simulink library "lithium_ion_battery"  (R2026a)
settings: Solver=VariableStepAuto
undefined symbols (not defined in the file): param, q1Kalman, q2Kalman, q3Kalman, rKalman, tc, ts_battery
libraries: nesl_utility x5, fl_lib x4, lithium_ion_cell_lib x1, simulink x1
settings Model: Creator=dbagn  LastModifiedBy=d.bagnara

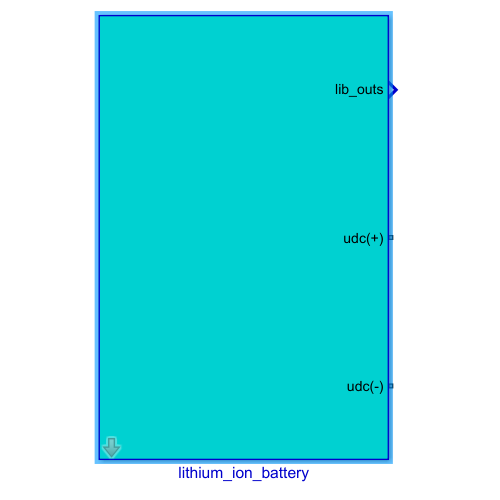
[thumbnail: Simulink's stored preview of the top-level diagram]
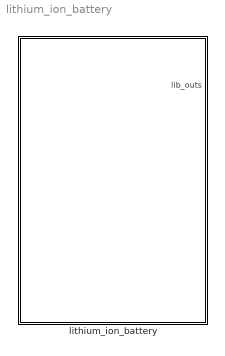
== system lithium_ion_battery ==
  lithium_ion_battery : Subsystem  mask{Q=50, number_of_cells=346, E_1=-1.031, E0=3.485, E1=0, E2=0, E3=0, Elog=-0.05, R0=0.0035, R1=0.0035, C1=0.5, M=125, alpha=35, soc_init=0.85, ts_battery=ts_battery, q1Kalman=q1Kalman, q2Kalman=q2Kalman, q3Kalman=q3Kalman, rKalman=rKalman, tc=tc, enable_white_noise_m=0, battery_voltage_init_m=param.battery.nominal_battery_voltage_1}
      mask prompts: Q "Nominal Charge Capacity (Ah)"; number_of_cells "Number of Cells"; E_1 "E_1 (V)"; E0 "E0 (V)"; E1 "E1 (V)"; E2 "E2 (V)"; E3 "E3 (V)"; Elog "Elog (V)"; R0 "R0 (Ohm)"; R1 "R1 (Ohm)"; C1 "C1 (F)"; M "Hysteresis coefficient (V)"; soc_init "State of Charge Init (pu)"; ts_battery "Sampling Time BESS"

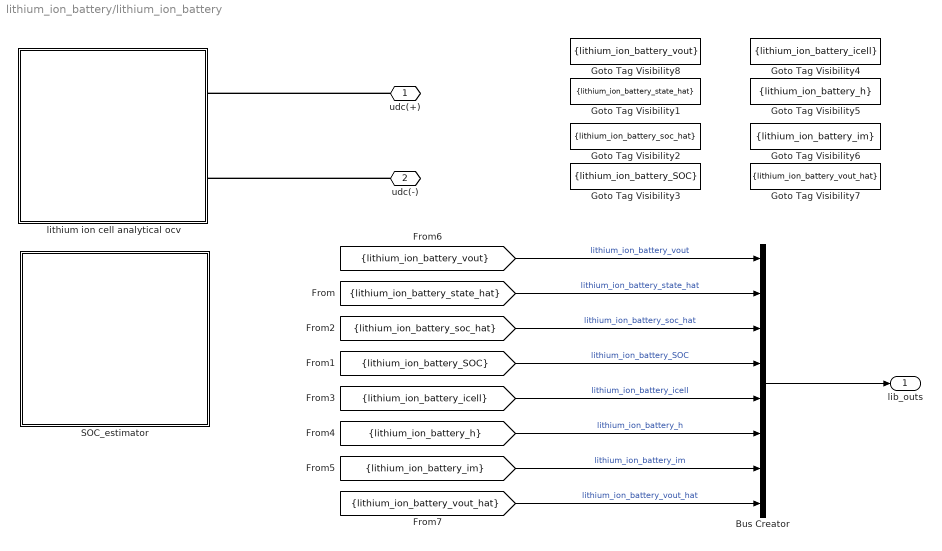
== system lithium_ion_battery/lithium_ion_battery ==
  Bus Creator : BusCreator  Inputs=8
  Goto Tag Visibility1 : GotoTagVisibility  GotoTag=lithium_ion_battery_state_hat
  Goto Tag Visibility2 : GotoTagVisibility  GotoTag=lithium_ion_battery_soc_hat
  Goto Tag Visibility3 : GotoTagVisibility  GotoTag=lithium_ion_battery_SOC
  Goto Tag Visibility4 : GotoTagVisibility  GotoTag=lithium_ion_battery_icell
  Goto Tag Visibility5 : GotoTagVisibility  GotoTag=lithium_ion_battery_h
  Goto Tag Visibility6 : GotoTagVisibility  GotoTag=lithium_ion_battery_im
  Goto Tag Visibility7 : GotoTagVisibility  GotoTag=lithium_ion_battery_vout_hat
  Goto Tag Visibility8 : GotoTagVisibility  GotoTag=lithium_ion_battery_vout
  SOC_estimator : Subsystem
  lithium ion cell analytical ocv : Subsystem
  udc(+) : PMIOPort  Side=Right
  udc(-) : PMIOPort  Port=2  Side=Right
  lib_outs : Outport
  wires:
  [lithium_ion_battery_im] -> Bus Creator/7  "lithium_ion_battery_im"
  [lithium_ion_battery_h] -> Bus Creator/6  "lithium_ion_battery_h"
  [lithium_ion_battery_icell] -> Bus Creator/5  "lithium_ion_battery_icell"
  [lithium_ion_battery_SOC] -> Bus Creator/4  "lithium_ion_battery_SOC"
  [lithium_ion_battery_soc_hat] -> Bus Creator/3  "lithium_ion_battery_soc_hat"
  [lithium_ion_battery_state_hat] -> Bus Creator/2  "lithium_ion_battery_state_hat"
  [lithium_ion_battery_vout] -> Bus Creator/1  "lithium_ion_battery_vout"
  Bus Creator/1 -> lib_outs/1
  [lithium_ion_battery_vout_hat] -> Bus Creator/8  "lithium_ion_battery_vout_hat"
  connections:
  udc(-)/RConn1 -- lithium ion cell analytical ocv/RConn2
  udc(+)/RConn1 -- lithium ion cell analytical ocv/RConn1

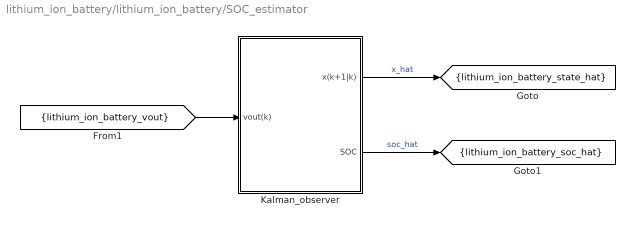
== system lithium_ion_battery/lithium_ion_battery/SOC_estimator ==
  Kalman_observer : Subsystem
  tag scope: lithium_ion_battery_soc_hat=scoped, lithium_ion_battery_state_hat=scoped
  wires:
  [lithium_ion_battery_vout] -> Kalman_observer/1(vout(k))
  Kalman_observer/1(x(k+1|k)) -> [lithium_ion_battery_state_hat]  "x_hat"
  Kalman_observer/2(SOC) -> [lithium_ion_battery_soc_hat]  "soc_hat"

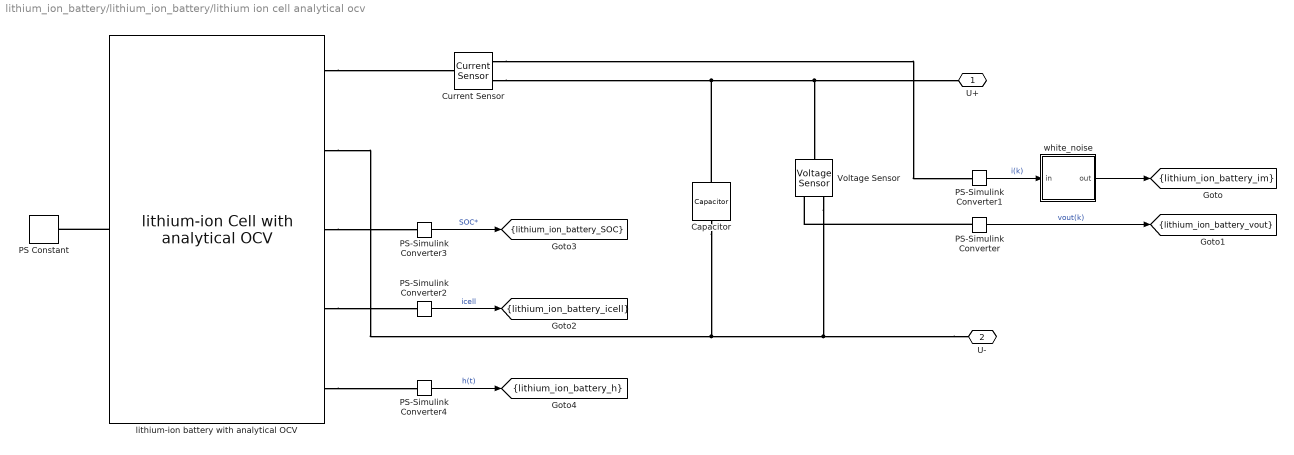
== system lithium_ion_battery/lithium_ion_battery/lithium ion cell analytical ocv ==
  Capacitor : fl_lib/Electrical/Electrical Elements/Capacitor  c=1e-3 F  r=1e-6 Ohm  g=0 1/Ohm  i_specify=off  i_priority=None  i=0 A  i_nominal_specify=off  i_nominal_value=1  i_nominal_unit=A  v_specify=off  v_priority=None  v=0 V  v_nominal_specify=off  v_nominal_value=1  v_nominal_unit=V  vc_specify=on  vc_priority=High  vc=battery_voltage_init_m V  vc_nominal_specify=off  vc_nominal_value=1  vc_nominal_unit=V
  Current Sensor : fl_lib/Electrical/Electrical Sensors/Current Sensor
  PS Constant : fl_lib/Physical Signals/Sources/PS Constant  constant=298.15 K
  PS-Simulink Converter{,1..4} (5 alike) : nesl_utility/PS-Simulink Converter  PhysicalDomain=network_engine_domain  SubClassName=ps_output  LeftPortType=input  RightPortType=output  PseudoPeriodic=off  Frequencies=[]  VectorFormat=1-D array  Unit=inherit  AffineConversion=off
  Voltage Sensor : fl_lib/Electrical/Electrical Sensors/Voltage Sensor
  lithium-ion battery with analytical OCV : lithium_ion_cell_lib/lithium-ion Cell with analytical OCV  Qcell=Q hr*A  N=number_of_cells  E_1=E_1 V  E0=E0 V  E1=E1 V  E2=E2 V  E3=E3 V  Elog=Elog V  R0=R0 Ohm  R1=R1 Ohm  C1=C1 F  M=M V  alpha=alpha  u_specify=off  u_priority=High  u=Vdc V  u_nominal_specify=off  u_nominal_value=1  u_nominal_unit=V  u_ocv_specify=off  u_ocv_priority=High  u_ocv=Vdc V  u_ocv_nominal_specify=off  u_ocv_nominal_value=1  u_ocv_nominal_unit=V  icell_specify=off  icell_priority=None  icell=0 A  icell_nominal_specify=off  icell_nominal_value=1  icell_nominal_unit=A  i_r1_specify=off  i_r1_priority=None  i_r1=0 A  i_r1_nominal_specify=off  i_r1_nominal_value=1  i_r1_nominal_unit=A  z_specify=on  z_priority=High  z=soc_init  z_nominal_specify=off  z_nominal_value=1  z_nominal_unit=1  h_specify=off  h_priority=High  h=0  h_nominal_specify=off  h_nominal_value=1  h_nominal_unit=1
  white_noise : Subsystem
  U+ : PMIOPort  Side=Right
  U- : PMIOPort  Port=2  Side=Right
  tag scope: lithium_ion_battery_SOC=scoped, lithium_ion_battery_h=scoped, lithium_ion_battery_icell=scoped, lithium_ion_battery_im=scoped, lithium_ion_battery_vout=scoped
  wires:
  PS-Simulink Converter/1 -> [lithium_ion_battery_vout]  "vout(k)"
  PS-Simulink Converter1/1 -> white_noise/1(in)  "i(k)"
  white_noise/1(out) -> [lithium_ion_battery_im]
  PS-Simulink Converter4/1 -> [lithium_ion_battery_h]  "h(t)"
  PS-Simulink Converter2/1 -> [lithium_ion_battery_icell]  "icell"
  PS-Simulink Converter3/1 -> [lithium_ion_battery_SOC]  "SOC*"
  connections:
  lithium-ion battery with analytical OCV/LConn1 -- PS Constant/RConn1
  PS-Simulink Converter/LConn1 -- Voltage Sensor/RConn1
  Current Sensor/RConn2 -- Capacitor/LConn1 -- U+/RConn1 -- Voltage Sensor/LConn1
  U-/RConn1 -- Capacitor/RConn1 -- lithium-ion battery with analytical OCV/RConn2 -- Voltage Sensor/RConn2
  Current Sensor/RConn1 -- PS-Simulink Converter1/LConn1
  lithium-ion battery with analytical OCV/RConn1 -- Current Sensor/LConn1
  lithium-ion battery with analytical OCV/RConn3 -- PS-Simulink Converter3/LConn1
  lithium-ion battery with analytical OCV/RConn4 -- PS-Simulink Converter2/LConn1
  lithium-ion battery with analytical OCV/RConn5 -- PS-Simulink Converter4/LConn1

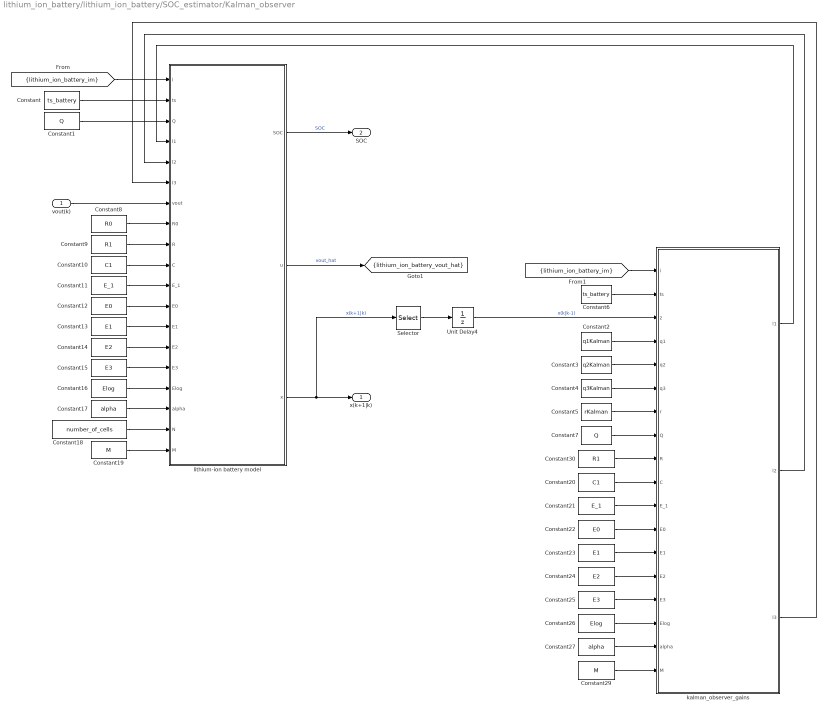
== system lithium_ion_battery/lithium_ion_battery/SOC_estimator/Kalman_observer ==
  vout(k) : Inport
  Constant : Constant  Value=ts_battery
  Constant1 : Constant  Value=Q
  Constant10 : Constant  Value=C1
  Constant11 : Constant  Value=E_1
  Constant12 : Constant  Value=E0
  Constant13 : Constant  Value=E1
  Constant14 : Constant  Value=E2
  Constant15 : Constant  Value=E3
  Constant16 : Constant  Value=Elog
  Constant17 : Constant  Value=alpha
  Constant18 : Constant  Value=number_of_cells
  Constant19 : Constant  Value=M
  Constant2 : Constant  Value=q1Kalman
  Constant20 : Constant  Value=C1
  Constant21 : Constant  Value=E_1
  Constant22 : Constant  Value=E0
  Constant23 : Constant  Value=E1
  Constant24 : Constant  Value=E2
  Constant25 : Constant  Value=E3
  Constant26 : Constant  Value=Elog
  Constant27 : Constant  Value=alpha
  Constant29 : Constant  Value=M
  Constant3 : Constant  Value=q2Kalman
  Constant30 : Constant  Value=R1
  Constant4 : Constant  Value=q3Kalman
  Constant5 : Constant  Value=rKalman
  Constant6 : Constant  Value=ts_battery
  Constant7 : Constant  Value=Q
  Constant8 : Constant  Value=R0
  Constant9 : Constant  Value=R1
  Selector : Selector  InputPortWidth=3  IndexOptions=Index vector (dialog)  Indices=1  OutputSizes=1
  Unit Delay4 : UnitDelay  SampleTime=ts_battery
  kalman_observer_gains : MATLAB Function  TreatAsAtomicUnit=on  SystemSampleTime=ts_battery
  lithium-ion battery model : MATLAB Function  TreatAsAtomicUnit=on  SystemSampleTime=ts_battery
  x(k+1|k) : Outport
  SOC : Outport  Port=2
  tag scope: lithium_ion_battery_vout_hat=scoped
  wires:
  lithium-ion battery model/2(u) -> [lithium_ion_battery_vout_hat]  "vout_hat"
  vout(k)/1 -> lithium-ion battery model/7(vout)
  lithium-ion battery model/3(x) -> Selector/1, x(k+1|k)/1  "x(k+1|k)"
  kalman_observer_gains/2(l2) -> lithium-ion battery model/5(l2)
  Constant6/1 -> kalman_observer_gains/2(ts)
  lithium-ion battery model/1(SOC) -> SOC/1  "SOC"
  Constant7/1 -> kalman_observer_gains/8(Q)
  kalman_observer_gains/3(l3) -> lithium-ion battery model/6(l3)
  Constant1/1 -> lithium-ion battery model/3(Q)
  Constant5/1 -> kalman_observer_gains/7(r)
  [lithium_ion_battery_im] -> kalman_observer_gains/1(i)
  Constant4/1 -> kalman_observer_gains/6(q3)
  Constant2/1 -> kalman_observer_gains/4(q1)
  kalman_observer_gains/1(l1) -> lithium-ion battery model/4(l1)
  Constant/1 -> lithium-ion battery model/2(ts)
  Constant3/1 -> kalman_observer_gains/5(q2)
  Unit Delay4/1 -> kalman_observer_gains/3(z)  "x(k|k-1)"
  Selector/1 -> Unit Delay4/1
  [lithium_ion_battery_im] -> lithium-ion battery model/1(i)
  Constant18/1 -> lithium-ion battery model/18(N)
  Constant8/1 -> lithium-ion battery model/8(R0)
  Constant9/1 -> lithium-ion battery model/9(R)
  Constant10/1 -> lithium-ion battery model/10(C)
  Constant11/1 -> lithium-ion battery model/11(E_1)
  Constant12/1 -> lithium-ion battery model/12(E0)
  Constant13/1 -> lithium-ion battery model/13(E1)
  Constant14/1 -> lithium-ion battery model/14(E2)
  Constant15/1 -> lithium-ion battery model/15(E3)
  Constant16/1 -> lithium-ion battery model/16(Elog)
  Constant17/1 -> lithium-ion battery model/17(alpha)
  Constant19/1 -> lithium-ion battery model/19(M)
  Constant29/1 -> kalman_observer_gains/18(M)
  Constant27/1 -> kalman_observer_gains/17(alpha)
  Constant26/1 -> kalman_observer_gains/16(Elog)
  Constant25/1 -> kalman_observer_gains/15(E3)
  Constant24/1 -> kalman_observer_gains/14(E2)
  Constant23/1 -> kalman_observer_gains/13(E1)
  Constant22/1 -> kalman_observer_gains/12(E0)
  Constant21/1 -> kalman_observer_gains/11(E_1)
  Constant20/1 -> kalman_observer_gains/10(C)
  Constant30/1 -> kalman_observer_gains/9(R)

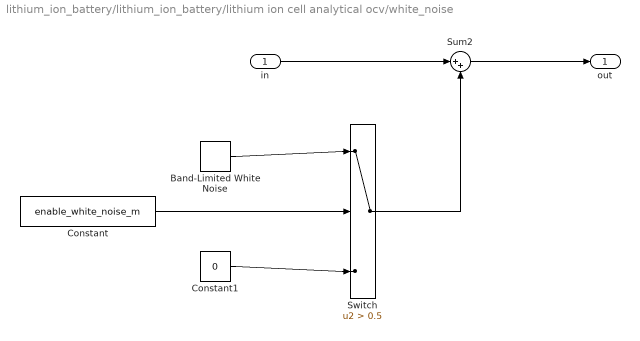
== system lithium_ion_battery/lithium_ion_battery/lithium ion cell analytical ocv/white_noise ==
  in : Inport
  Band-Limited White Noise : simulink/Sources/Band-Limited White Noise  Cov=tc  Ts=tc  seed=[23341]
  Constant : Constant  Value=enable_white_noise_m
  Constant1 : Constant  Value=0
  Sum2 : Sum  Inputs=|++
  Switch : Switch  Criteria=u2 > Threshold  Threshold=0.5  SaturateOnIntegerOverflow=off  InputSameDT=off
  out : Outport
  wires:
  Sum2/1 -> out/1
  in/1 -> Sum2/1
  Band-Limited White Noise/1 -> Switch/1
  Constant/1 -> Switch/2
  Constant1/1 -> Switch/3
  Switch/1 -> Sum2/2

== matlab function lithium_ion_battery/SOC_estimator/Kalman_observer/kalman_observer_gains ==
  data: i input; ts input; l1 output; z input; q1 input; q2 input; q3 input; r input; Q input; l2 output; l3 output; R input; C input; E_1 input; E0 input; E1 input; E2 input; E3 input; Elog input; alpha input; M input
function [l1,l2,l3] = EKF(i,ts,z,q1,q2,q3,r,Q, R, C, E_1, E0, E1, E2, E3, Elog, alpha, M)

    persistent  p11 p12 p13 p21 p22 p23 p31 p32 p33

    if isempty(p11)
        p11 = q1;
        p12 = 0;
        p13 = 0;
        p21 = 0;
        p22 = q2;
        p23 = 0;
        p31 = 0;
        p32 = 0;
        p33 = q3;
    end

    a11 = 1;
    a12 = 0;
    a13 = 0;
    a21 = 0;
    a22 = exp(-ts/(R*C));
    a23 = 0;
    a31 = 0;
    a32 = 0;
    a33 = abs(exp(-i*ts/Q));

    c1 = -alpha*E_1*abs(exp(-alpha*z)) + E1 + 2*E2*z + 3*E3*z^2 - Elog/(1-z+ts);
    c2 = -R;
    c3 = M;
    
    p11_pr = a11*(a11*p11 + a12*p21 + a13*p31) + a12*(a11*p12 + a12*p22 + a13*p32) + a13*(a11*p13 + a12*p23 + a13*p33) + q1;

    p12_pr = a21*(a11*p11 + a12*p21 + a13*p31) + a22*(a11*p12 + a12*p22 + a13*p32) + a23*(a11*p13 + a12*p23 + a13*p33);

    p13_pr = a31*(a11*p11 + a12*p21 + a13*p31) + a32*(a11*p12 + a12*p22 + a13*p32) + a33*(a11*p13 + a12*p23 + a13*p33);

    p21_pr = a11*(a21*p11 + a22*p21 + a23*p31) + a12*(a21*p12 + a22*p22 + a23*p32) + a13*(a21*p13 + a22*p23 + a23*p33);

    p22_pr = a21*(a21*p11 + a22*p21 + a23*p31) + a22*(a21*p12 + a22*p22 + a23*p32) + a23*(a21*p13 + a22*p23 + a23*p33) + q2;

    p23_pr = a31*(a21*p11 + a22*p21 + a23*p31) + a32*(a21*p12 + a22*p22 + a23*p32) + a33*(a21*p13 + a22*p23 + a23*p33);

    p31_pr = a11*(a31*p11 + a32*p21 + a33*p31) + a12*(a31*p12 + a32*p22 + a33*p32) + a13*(a31*p13 + a32*p23 + a33*p33);

    p32_pr = a21*(a31*p11 + a32*p21 + a33*p31) + a22*(a31*p12 + a32*p22 + a33*p32) + a23*(a31*p13 + a32*p23 + a33*p33);

    p33_pr = a31*(a31*p11 + a32*p21 + a33*p31) + a32*(a31*p12 + a32*p22 + a33*p32) + a33*(a31*p13 + a32*p23 + a33*p33) + q3;

    den = c1*(c1*p11 + c2*p21 + c3*p31) + c2*(c1*p12 + c2*p22 + c3*p32) + c3*(c1*p13 + c2*p23 + c3*p33) + r;
 
    l1 = (c1*p11 + c2*p12 + c3*p13)/den;
    l2 = (c1*p21 + c2*p22 + c3*p23)/den;
    l3 = (c1*p31 + c2*p32 + c3*p33)/den;
    
    p11 = (1 - c1*l1)*p11_pr - c2*l1*p21_pr - c3*l1*p31_pr;
    
    p12 = (1 - c1*l1)*p12_pr - c2*l1*p22_pr - c3*l1*p32_pr;
    
    p13 = (1 - c1*l1)*p13_pr - c2*l1*p23_pr - c3*l1*p33_pr;
    
    p21 = -c1*l2*p11_pr + (1 - c2*l2)*p21_pr - c3*l2*p31_pr;
    
    p22 = -c1*l2*p12_pr + (1 - c2*l2)*p22_pr - c3*l2*p32_pr;
    
    p23 = -c1*l2*p13_pr + (1 - c2*l2)*p23_pr - c3*l2*p33_pr;
    
    p31 = -c1*l3*p11_pr - c2*l3*p21_pr + (1 - c3*l3)*p31_pr;
    
    p32 = -c1*l3*p12_pr - c2*l3*p22_pr + (1 - c3*l3)*p32_pr;
    
    p33 = -c1*l3*p13_pr - c2*l3*p23_pr + (1 - c3*l3)*p33_pr;
end

== matlab function lithium_ion_battery/SOC_estimator/Kalman_observer/lithium-ion battery model ==
  data: i input; SOC output; u output; ts input; Q input; l1 input; l2 input; l3 input; vout input; x output; R0 input; R input; C input; E_1 input; E0 input; E1 input; E2 input; E3 input; Elog input; alpha input; N input; M input
function [SOC, u, x] = lithium_ion_battery(i,ts,Q,l1,l2,l3,vout, R0, R,C, E_1, E0, E1, E2, E3, Elog, alpha, N, M)

    persistent z_po ir_po h_po vout_hat

    if isempty(z_po)
        ir_po = 0;
        h_po = 0;
        z_po = 0.5;        
    end      
        
        Q = Q * 3600; 
        z_pr = z_po - ts/Q*i ;
    
        ir_pr = exp(-ts/(R*C))*ir_po + (1-exp(-ts/(R*C)))*i;

        h_pr = exp(-abs(i)*ts/Q)*h_po - (1-exp(-abs(i)*ts/Q))*sign(i);
        
        OCV = E_1*exp(-z_pr*alpha) + E0 + E1*z_pr + E2*z_pr^2 + E3*z_pr^3 + Elog*log(abs(1-z_pr+ts));
        
        vout_hat = OCV*N + M*h_pr - R*ir_pr - R0*i;
        
        z_po = z_pr + l1*(vout - vout_hat);
        ir_po = ir_pr + l2*(vout - vout_hat);
        h_po = h_pr + l3*(vout - vout_hat);
        u = vout_hat;
        
        x = [z_po; ir_po; h_po];

    SOC = z_po;
end
